simulink library "frame_switch_block"  (R2025b)
settings: Solver=VariableStepAuto  StartTime=0.0  StopTime=10.0  RelTol=1e-3
settings Model: Creator=Ashwin  LastModifiedBy=Ashwin

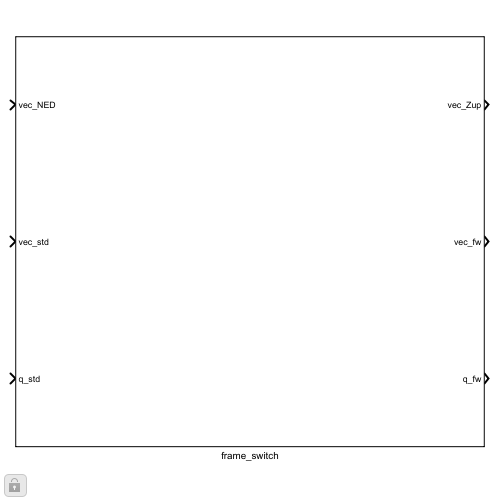
[thumbnail: Simulink's stored preview of the top-level diagram]
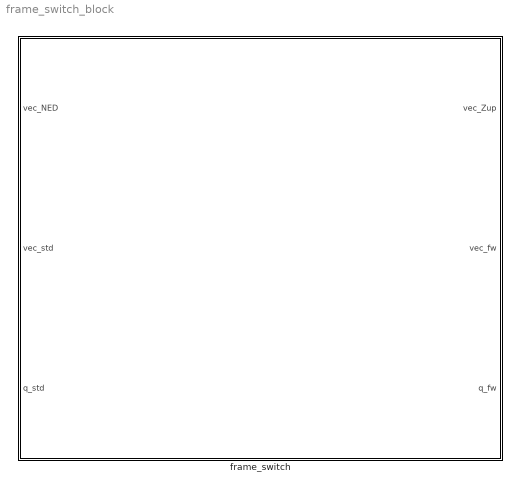
== system frame_switch_block ==
  frame_switch : Subsystem

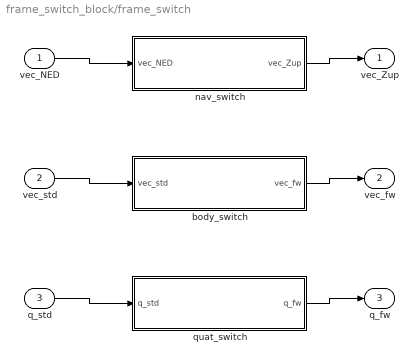
== system frame_switch_block/frame_switch ==
  vec_NED : Inport
  vec_std : Inport  Port=2
  q_std : Inport  Port=3
  body_switch : MATLAB Function  TreatAsAtomicUnit=on
  nav_switch : MATLAB Function  TreatAsAtomicUnit=on
  quat_switch : MATLAB Function  TreatAsAtomicUnit=on
  vec_Zup : Outport
  vec_fw : Outport  Port=2
  q_fw : Outport  Port=3
  wires:
  vec_NED/1 -> nav_switch/1(vec_NED)
  nav_switch/1(vec_Zup) -> vec_Zup/1
  vec_std/1 -> body_switch/1(vec_std)
  body_switch/1(vec_fw) -> vec_fw/1
  q_std/1 -> quat_switch/1(q_std)
  quat_switch/1(q_fw) -> q_fw/1

== matlab function frame_switch_block/frame_switch/nav_switch ==
  data: vec_NED input; vec_Zup output
function vec_Zup = nav_switch(vec_NED)

== matlab function frame_switch_block/frame_switch/quat_switch ==
  data: q_std input; q_fw output
function q_fw = quat_switch(q_std)

== matlab function frame_switch_block/frame_switch/body_switch ==
  data: vec_std input; vec_fw output
function vec_fw = body_switch(vec_std)
